simulink model "Robot_Controller"  (R2025b)
settings: Solver=FixedStepAuto  StartTime=0.0  StopTime=10.0  RelTol=1e-3
settings Model: Creator=Rhythm  LastModifiedBy=Rhythm
settings RTWCC: GenCodeOnly=on

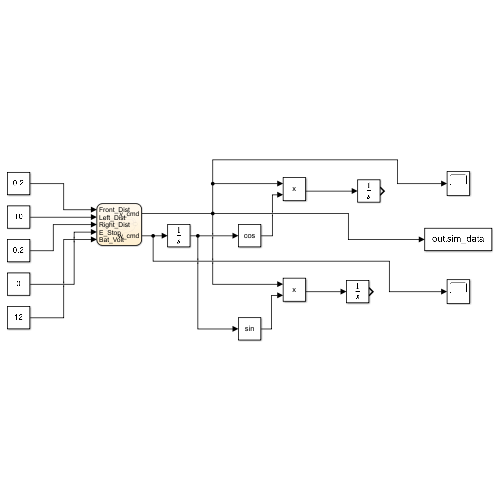
[thumbnail: Simulink's stored preview of the top-level diagram]
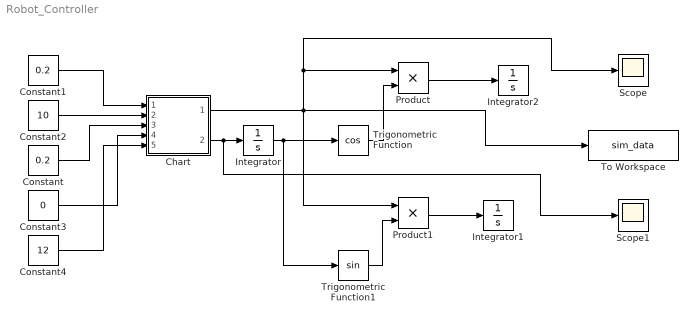
== system Robot_Controller ==
  Chart : Stateflow chart  TreatAsAtomicUnit=on
  Constant : Constant  Value=0.2
  Constant1 : Constant  Value=0.2
  Constant2 : Constant  Value=10
  Constant3 : Constant  Value=0
  Constant4 : Constant  Value=12
  Integrator : Integrator
  Integrator1 : Integrator
  Integrator2 : Integrator
  Product : Product
  Product1 : Product
  Scope : Scope
      settings: ActiveDisplayYMinimum=-1.2105703065542321  ActiveDisplayYMaximum=2.0165863105062192
  Scope1 : Scope
      settings: ActiveDisplayYMinimum=-8.6219527671062828  ActiveDisplayYMaximum=12.556271445242135
  To Workspace : ToWorkspace  VariableName=sim_data  SampleTime=-1
  Trigonometric Function : Trigonometry  Operator=cos
  Trigonometric Function1 : Trigonometry
  wires:
  Constant/1 -> Chart/3(Right_Dist)
  Constant2/1 -> Chart/2(Left_Dist)
  Chart/2(w_cmd) -> Integrator/1, Scope1/1
  Integrator/1 -> Trigonometric Function/1, Trigonometric Function1/1
  Chart/1(v_cmd) -> Scope/1, Product/1, To Workspace/1, Product1/1
  Trigonometric Function/1 -> Product/2
  Product/1 -> Integrator2/1
  Trigonometric Function1/1 -> Product1/2
  Product1/1 -> Integrator1/1
  Constant1/1 -> Chart/1(Front_Dist)
  Constant3/1 -> Chart/4(E_Stop)
  Constant4/1 -> Chart/5(Bat_Volt)

== stateflow chart Robot_Controller/Chart ==
  state MoveForward
    entry:
    v_cmd = 0.5;
    w_cmd = 0;
  state Stop
    entry:
    v_cmd = 0;
    w_cmd = 0;
  state TurnLeft
    entry:
    v_cmd = 0;
    w_cmd = 0.5;
  state TurnRight
    entry:
    v_cmd = 0;
    w_cmd = -0.5;
  state Emergency
    entry:
    v_cmd = 0;
    w_cmd = 0;
  Stop -> Emergency [order 3] : [E_Stop == 1 || Bat_Volt < 10]
  TurnLeft -> MoveForward [order 1] : [Front_Dist > 0.8]
  TurnLeft -> Emergency [order 2] : [E_Stop == 1 || Bat_Volt < 10]
  (default) -> MoveForward
  Stop -> TurnLeft [order 1] : [Right_Dist < 0.5 && Left_Dist > 0.5]
  TurnRight -> Emergency [order 2] : [E_Stop == 1 || Bat_Volt < 10]
  MoveForward -> Stop [order 1] : [Front_Dist < 0.5]
  Emergency -> Stop : [E_Stop == 0]
  TurnRight -> MoveForward [order 1] : [Front_Dist > 0.8]
  MoveForward -> Emergency [order 2] : [E_Stop == 1 || Bat_Volt < 10]
  Stop -> TurnRight [order 2] : [Left_Dist < 0.5 && Right_Dist > 0.5]
  data: Front_Dist input; Left_Dist input; Right_Dist input; v_cmd output; w_cmd output; E_Stop input; Bat_Volt input
